simulink model "Reactor_Gp1"  (Simulink 7.5)
settings: Solver=ode4  StartTime=0.0  StopTime=20  FixedStep=0.01  RelTol=1e-3
values from neighbouring files (symbols this model uses):
  K = 0.3199    [Ex14Gp1.m]    (also in Ex14Gp2.m)
  Kc = 1/K*(a1*(L/T)^b1+c1)    [Jrd3Deg_PID1tuning.m]    (also in Jrd3Degd_PID1tuning.m; MaxSenPID.m = pid(1))
  Ln = 0.5289    [Ex14Gp1.m]    (also in Ex14Gp2.m)
  T = 0.6238    [Ex14Gp1.m]    (also in Ex14Gp2.m)
  Td = T*(a3*(L/T)^b3+c3)    [Jrd3Deg_PID1tuning.m]    (also in Jrd3Degd_PID1tuning.m; MaxSenPID.m = pid(3))
  Ti = T*(a2*(L/T)^b2+c2)    [Jrd3Deg_PID1tuning.m]    (also in Jrd3Degd_PID1tuning.m; MaxSenPID.m = pid(2))
settings Model: Creator=Orlo  LastModifiedBy=oarrieta
settings OptimizationCC: InlineInvariantSignals=on  InitFltsAndDblsToZero=on
settings DebuggingCC: SaveWithParameterizedLinksMsg=none  SignalResolutionControl=TryResolveAllWithWarning  MultiTaskDSMMsg=warning  MultiTaskCondExecSysMsg=none  StrictBusMsg=None
settings RTWCC: IncludeERTFirstTime=on
settings GRTTargetCC: TargetFcnLib=ansi_tfl_tmw.mat

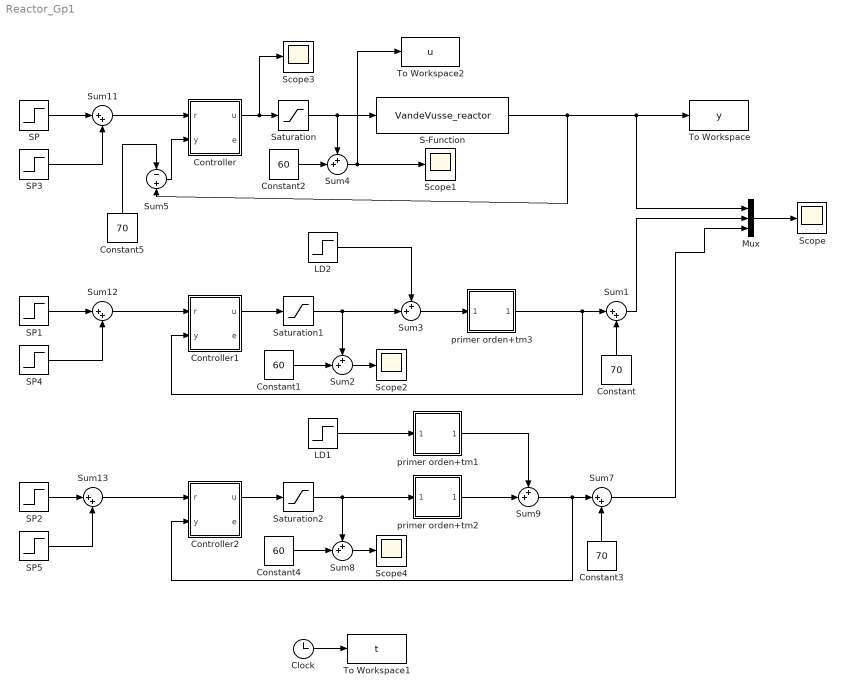
== system Reactor_Gp1 ==
  Clock : Clock
      settings: Decimation=10
  Constant : Constant  Value=70  OutDataType=sfix(16)  OutScaling=2^0
  Constant1 : Constant  Value=60  OutDataType=sfix(16)  OutScaling=2^0
  Constant2 : Constant  Value=60  OutDataType=sfix(16)  OutScaling=2^0
  Constant3 : Constant  Value=70  OutDataType=sfix(16)  OutScaling=2^0
  Constant4 : Constant  Value=60  OutDataType=sfix(16)  OutScaling=2^0
  Constant5 : Constant  Value=70  OutDataType=sfix(16)  OutScaling=2^0
  Controller : Subsystem  mask{Kc=Kc, Ti=Ti, Td=Td, b=1}
      mask prompts: Kc "Controller Gain - Kc"; Ti "Integral Time Constant - Ti"; Td "Derivative Time Constant - Td"; b "Set-point Weight - beta"
      mask Display:
      | disp('PID')
      | port_label('output',1,'u')
      | port_label('output',2,'e')
      | port_label('input',1,'r')
      | port_label('input',2,'y')
  Controller1 : Subsystem  mask{Kc=Kc, Ti=Ti, Td=Td, b=1}
      mask prompts: Kc "Controller Gain - Kc"; Ti "Integral Time Constant - Ti"; Td "Derivative Time Constant - Td"; b "Set-point Weight - beta"
      mask Display:
      | disp('PID')
      | port_label('output',1,'u')
      | port_label('output',2,'e')
      | port_label('input',1,'r')
      | port_label('input',2,'y')
  Controller2 : Subsystem  mask{Kc=Kc, Ti=Ti, Td=Td, b=1}
      mask prompts: Kc "Controller Gain - Kc"; Ti "Integral Time Constant - Ti"; Td "Derivative Time Constant - Td"; b "Set-point Weight - beta"
      mask Display:
      | disp('PID')
      | port_label('output',1,'u')
      | port_label('output',2,'e')
      | port_label('input',1,'r')
      | port_label('input',2,'y')
  LD1 : Step  Time=10  SampleTime=0
  LD2 : Step  Time=10  SampleTime=0
  Mux : Mux  Inputs=3
  S-Function : S-Function  FunctionName=VandeVusse_reactor  Parameters=2.9175, 1.10  EnableBusSupport=off
  SP : Step  After=-10  SampleTime=0
  SP1 : Step  After=-10  SampleTime=0
  SP2 : Step  After=-10  SampleTime=0
  SP3 : Step  Time=15  After=5  SampleTime=0
  SP4 : Step  Time=20  After=5  SampleTime=0
  SP5 : Step  Time=20  After=5  SampleTime=0
  Saturation : Saturate  UpperLimit=40  LowerLimit=-60
  Saturation1 : Saturate  UpperLimit=40  LowerLimit=-60
  Saturation2 : Saturate  UpperLimit=40  LowerLimit=-60
  Scope{,1..4} (5 alike) : Scope
      Scope settings: YMin=54  YMax=74
      Scope1 settings: YMin=77  YMax=97
      Scope2 settings: YMin=65  YMax=90  SaveName=ScopeData2
      Scope3 settings: YMin=87.6517  YMax=87.6518  SaveName=ScopeData3
      Scope4 settings: YMin=65  YMax=90  SaveName=ScopeData4
  Sum{1,7,11..13} (5 alike) : Sum  Inputs=|++  OutDataType=sfix(16)  OutScaling=2^0  SaturateOnIntegerOverflow=on
  Sum{2..4,8..9} (5 alike) : Sum  Inputs=++|  OutDataType=sfix(16)  OutScaling=2^0  SaturateOnIntegerOverflow=on
  Sum5 : Sum  Inputs=-|+  OutDataType=sfix(16)  OutScaling=2^0  SaturateOnIntegerOverflow=on
  To Workspace : ToWorkspace  VariableName=y  SampleTime=-1  SaveFormat=Array
  To Workspace1 : ToWorkspace  VariableName=t  SampleTime=-1  SaveFormat=Array
  To Workspace2 : ToWorkspace  VariableName=u  SampleTime=-1  SaveFormat=Array
  primer orden+tm1 : Subsystem  mask(Modelo de primer orden mas tiempo muerto){K=5.4624, T=0.6829, L=0.2209}
      mask prompts: K "Ganancia"; T "Constante de tiempo"; L "Retardo"
      mask help:
      | Introduzca el valor para los parametros de la constante de tiempo y del retardo para el sistema de primer orden con retardo
      | Gm(s)=exp(-Ls)/(1+Ts)
      mask Display: disp('Modelo')
  primer orden+tm2 : Subsystem  mask(Modelo de primer orden mas tiempo muerto){K=K, T=T, L=Ln}
      mask prompts: K "Ganancia"; T "Constante de tiempo"; L "Retardo"
      mask help:
      | Introduzca el valor para los parametros de la constante de tiempo y del retardo para el sistema de primer orden con retardo
      | Gm(s)=exp(-Ls)/(1+Ts)
      mask Display: disp('Modelo')
  primer orden+tm3 : Subsystem  mask(Modelo de primer orden mas tiempo muerto){K=K, T=T, L=Ln}
      mask prompts: K "Ganancia"; T "Constante de tiempo"; L "Retardo"
      mask help:
      | Introduzca el valor para los parametros de la constante de tiempo y del retardo para el sistema de primer orden con retardo
      | Gm(s)=exp(-Ls)/(1+Ts)
      mask Display: disp('Modelo')
  wires:
  S-Function/1 -> Mux/1, To Workspace/1, Sum5/2
  Controller/1(u) -> Saturation/1, Scope3/1
  Saturation/1 -> S-Function/1, Sum4/1
  LD2/1 -> Sum3/1
  Saturation1/1 -> Sum2/1, Sum3/2
  Controller1/1(u) -> Saturation1/1
  Constant/1 -> Sum1/2
  Mux/1 -> Scope/1
  Sum1/1 -> Mux/2
  Sum2/1 -> Scope2/1
  Constant1/1 -> Sum2/2
  Sum4/1 -> Scope1/1, To Workspace2/1
  Constant2/1 -> Sum4/2
  LD1/1 -> primer orden+tm1/1(In_1)
  primer orden+tm1/1(Out_1) -> Sum9/1
  primer orden+tm2/1(Out_1) -> Sum9/2
  Saturation2/1 -> Sum8/1, primer orden+tm2/1(In_1)
  Controller2/1(u) -> Saturation2/1
  Sum9/1 -> Sum7/1, Controller2/2(y)
  Constant3/1 -> Sum7/2
  Sum8/1 -> Scope4/1
  Constant4/1 -> Sum8/2
  Sum7/1 -> Mux/3
  Clock/1 -> To Workspace1/1
  SP/1 -> Sum11/1
  SP3/1 -> Sum11/2
  Sum11/1 -> Controller/1(r)
  SP1/1 -> Sum12/1
  Sum12/1 -> Controller1/1(r)
  SP4/1 -> Sum12/2
  SP2/1 -> Sum13/1
  Sum13/1 -> Controller2/1(r)
  SP5/1 -> Sum13/2
  primer orden+tm3/1(Out_1) -> Sum1/1, Controller1/2(y)
  Sum3/1 -> primer orden+tm3/1(In_1)
  Constant5/1 -> Sum5/1
  Sum5/1 -> Controller/2(y)

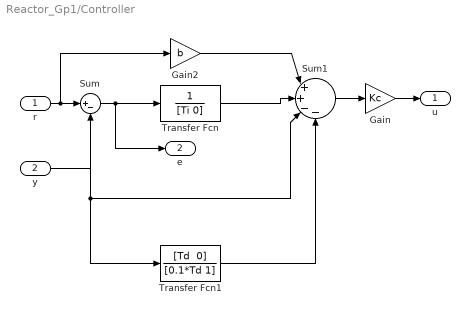
== system Reactor_Gp1/Controller ==
  r : Inport  OutDataType=sfix(16)  OutScaling=2^0
  y : Inport  Port=2  OutDataType=sfix(16)  OutScaling=2^0
  Gain : Gain  Gain=Kc  ParameterDataType=sfix(16)  ParameterScaling=2^0  OutDataType=sfix(16)  OutScaling=2^0  SaturateOnIntegerOverflow=on  OutDataTypeStr=Inherit: Same as input  ParamDataTypeStr=Inherit: Same as input
  Gain2 : Gain  Gain=b  ParameterDataType=sfix(16)  ParameterScaling=2^0  OutDataType=sfix(16)  OutScaling=2^0  SaturateOnIntegerOverflow=on  OutDataTypeStr=Inherit: Same as input  ParamDataTypeStr=Inherit: Same as input
  Sum : Sum  Inputs=|+-  OutDataType=sfix(16)  OutScaling=2^0  SaturateOnIntegerOverflow=on
  Sum1 : Sum  Inputs=|++--  OutDataType=sfix(16)  OutScaling=2^0  SaturateOnIntegerOverflow=on
  Transfer Fcn : TransferFcn  Denominator=[Ti 0]
  Transfer Fcn1 : TransferFcn  Numerator="[Td  0]"  Denominator=[0.1*Td 1]
  u : Outport  OutDataType=sfix(16)  OutScaling=2^0
  e : Outport  Port=2  OutDataType=sfix(16)  OutScaling=2^0
  wires:
  Transfer Fcn1/1 -> Sum1/4
  Gain2/1 -> Sum1/1
  Transfer Fcn/1 -> Sum1/2
  Gain/1 -> u/1
  y/1 -> Sum1/3, Sum/2, Transfer Fcn1/1
  r/1 -> Gain2/1, Sum/1
  Sum1/1 -> Gain/1
  Sum/1 -> Transfer Fcn/1, e/1

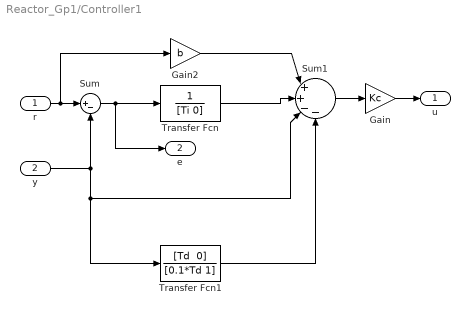
== system Reactor_Gp1/Controller1 ==
  r : Inport  OutDataType=sfix(16)  OutScaling=2^0
  y : Inport  Port=2  OutDataType=sfix(16)  OutScaling=2^0
  Gain : Gain  Gain=Kc  ParameterDataType=sfix(16)  ParameterScaling=2^0  OutDataType=sfix(16)  OutScaling=2^0  SaturateOnIntegerOverflow=on  OutDataTypeStr=Inherit: Same as input  ParamDataTypeStr=Inherit: Same as input
  Gain2 : Gain  Gain=b  ParameterDataType=sfix(16)  ParameterScaling=2^0  OutDataType=sfix(16)  OutScaling=2^0  SaturateOnIntegerOverflow=on  OutDataTypeStr=Inherit: Same as input  ParamDataTypeStr=Inherit: Same as input
  Sum : Sum  Inputs=|+-  OutDataType=sfix(16)  OutScaling=2^0  SaturateOnIntegerOverflow=on
  Sum1 : Sum  Inputs=|++--  OutDataType=sfix(16)  OutScaling=2^0  SaturateOnIntegerOverflow=on
  Transfer Fcn : TransferFcn  Denominator=[Ti 0]
  Transfer Fcn1 : TransferFcn  Numerator="[Td  0]"  Denominator=[0.1*Td 1]
  u : Outport  OutDataType=sfix(16)  OutScaling=2^0
  e : Outport  Port=2  OutDataType=sfix(16)  OutScaling=2^0
  wires:
  Transfer Fcn1/1 -> Sum1/4
  Gain2/1 -> Sum1/1
  Transfer Fcn/1 -> Sum1/2
  Gain/1 -> u/1
  y/1 -> Sum1/3, Sum/2, Transfer Fcn1/1
  r/1 -> Gain2/1, Sum/1
  Sum1/1 -> Gain/1
  Sum/1 -> Transfer Fcn/1, e/1

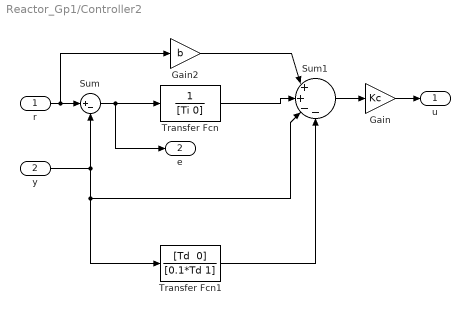
== system Reactor_Gp1/Controller2 ==
  r : Inport  OutDataType=sfix(16)  OutScaling=2^0
  y : Inport  Port=2  OutDataType=sfix(16)  OutScaling=2^0
  Gain : Gain  Gain=Kc  ParameterDataType=sfix(16)  ParameterScaling=2^0  OutDataType=sfix(16)  OutScaling=2^0  SaturateOnIntegerOverflow=on  OutDataTypeStr=Inherit: Same as input  ParamDataTypeStr=Inherit: Same as input
  Gain2 : Gain  Gain=b  ParameterDataType=sfix(16)  ParameterScaling=2^0  OutDataType=sfix(16)  OutScaling=2^0  SaturateOnIntegerOverflow=on  OutDataTypeStr=Inherit: Same as input  ParamDataTypeStr=Inherit: Same as input
  Sum : Sum  Inputs=|+-  OutDataType=sfix(16)  OutScaling=2^0  SaturateOnIntegerOverflow=on
  Sum1 : Sum  Inputs=|++--  OutDataType=sfix(16)  OutScaling=2^0  SaturateOnIntegerOverflow=on
  Transfer Fcn : TransferFcn  Denominator=[Ti 0]
  Transfer Fcn1 : TransferFcn  Numerator="[Td  0]"  Denominator=[0.1*Td 1]
  u : Outport  OutDataType=sfix(16)  OutScaling=2^0
  e : Outport  Port=2  OutDataType=sfix(16)  OutScaling=2^0
  wires:
  Transfer Fcn1/1 -> Sum1/4
  Gain2/1 -> Sum1/1
  Transfer Fcn/1 -> Sum1/2
  Gain/1 -> u/1
  y/1 -> Sum1/3, Sum/2, Transfer Fcn1/1
  r/1 -> Gain2/1, Sum/1
  Sum1/1 -> Gain/1
  Sum/1 -> Transfer Fcn/1, e/1

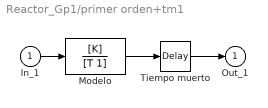
== system Reactor_Gp1/primer orden+tm1 ==
  In_1 : Inport  OutDataType=sfix(16)  OutScaling=2^0
  Modelo : TransferFcn  Numerator=[K]  Denominator=[T 1]
  Tiempo muerto : TransportDelay  DelayTime=L
  Out_1 : Outport  OutDataType=sfix(16)  OutScaling=2^0  InitialOutput=0
  wires:
  Modelo/1 -> Tiempo muerto/1
  In_1/1 -> Modelo/1
  Tiempo muerto/1 -> Out_1/1

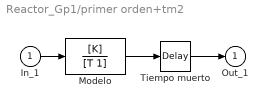
== system Reactor_Gp1/primer orden+tm2 ==
  In_1 : Inport  OutDataType=sfix(16)  OutScaling=2^0
  Modelo : TransferFcn  Numerator=[K]  Denominator=[T 1]
  Tiempo muerto : TransportDelay  DelayTime=L
  Out_1 : Outport  OutDataType=sfix(16)  OutScaling=2^0  InitialOutput=0
  wires:
  Modelo/1 -> Tiempo muerto/1
  In_1/1 -> Modelo/1
  Tiempo muerto/1 -> Out_1/1

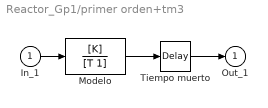
== system Reactor_Gp1/primer orden+tm3 ==
  In_1 : Inport  OutDataType=sfix(16)  OutScaling=2^0
  Modelo : TransferFcn  Numerator=[K]  Denominator=[T 1]
  Tiempo muerto : TransportDelay  DelayTime=L
  Out_1 : Outport  OutDataType=sfix(16)  OutScaling=2^0  InitialOutput=0
  wires:
  Modelo/1 -> Tiempo muerto/1
  In_1/1 -> Modelo/1
  Tiempo muerto/1 -> Out_1/1
